simulink model "Ld_Lq_realised_inverter"  (R2021b)
settings: Solver=ode23tb  StartTime=0.0  StopTime=0.05  MaxStep=1e-6  RelTol=1e-3  EnableMultiTasking=on
libraries: spsMosfetLib x6, spsCurrentMeasurementLib x5, spsRMSLib x5, spsVoltageMeasurementLib x4, spsSeriesRLCBranchLib x2, spsMeanLib x2, spsDCVoltageSourceLib x1, spsThreePhaseSeriesRLCBranchLib x1, simulink x1, spspowerguiLib x1
settings Model: SimulationMode=accelerator  Creator=Алексей  LastModifiedBy=Len_comp
settings SolverCC: ZeroCrossControl=DisableAll  ZeroCrossAlgorithm=Adaptive  AlgebraicLoopSolver=TrustRegion
settings DataIOCC: SaveFormat=Array  SaveOutput=off  SignalLogging=off  DSMLogging=off  SaveTime=off  ReturnWorkspaceOutputs=off
settings OptimizationCC: LifeSpan=inf
settings DebuggingCC: UnderspecifiedInitializationDetection=Classic  MergeDetectMultiDrivingBlocksExec=none  SolverPrmCheckMsg=warning  AllowSymbolicDim=off  SFUnexpectedBacktrackingDiag=warning  SFNoUnconditionalDefaultTransitionDiag=warning  SFExecutionAtInitializationDiag=none  SFMachineParentedDataDiag=warning  ArithmeticOperatorsInVariantConditions=warning
settings HardwareCC: ProdBitPerPointer=32  ProdBitPerSizeT=32  ProdBitPerPtrDiffT=32  ProdLargestAtomicFloat=None  ProdIntDivRoundTo=Undefined  ProdEndianess=Unspecified  ProdWordSize=32  ProdHWDeviceType=32-bit Generic
settings ModelReferenceCC: PropagateSignalLabelsOutOfModel=off
settings SFSimCC: SimUseLocalCustomCode=off  CustomCodeUndefinedFunction=UseInterfaceOnly
settings RTWCC: RTWUseLocalCustomCode=off
settings CodeAppCC: StateflowObjectComments=on
settings GRTTargetCC: TargetLangStandard=C89/C90 (ANSI)  RTWCAPISignals=on  RTWCAPIParams=on
settings ConfigComp: CovMetricSettings=dw  CovSaveCumulativeToWorkspaceVar=on  CovSaveSingleToWorkspaceVar=on  CovExternalEMLEnable=off  CovSFcnEnable=off
settings SimscapeCC: SimscapeNormalizeSystem=off

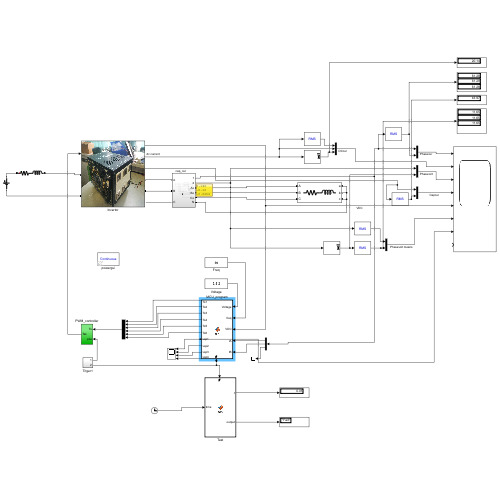
[thumbnail: Simulink's stored preview of the top-level diagram]
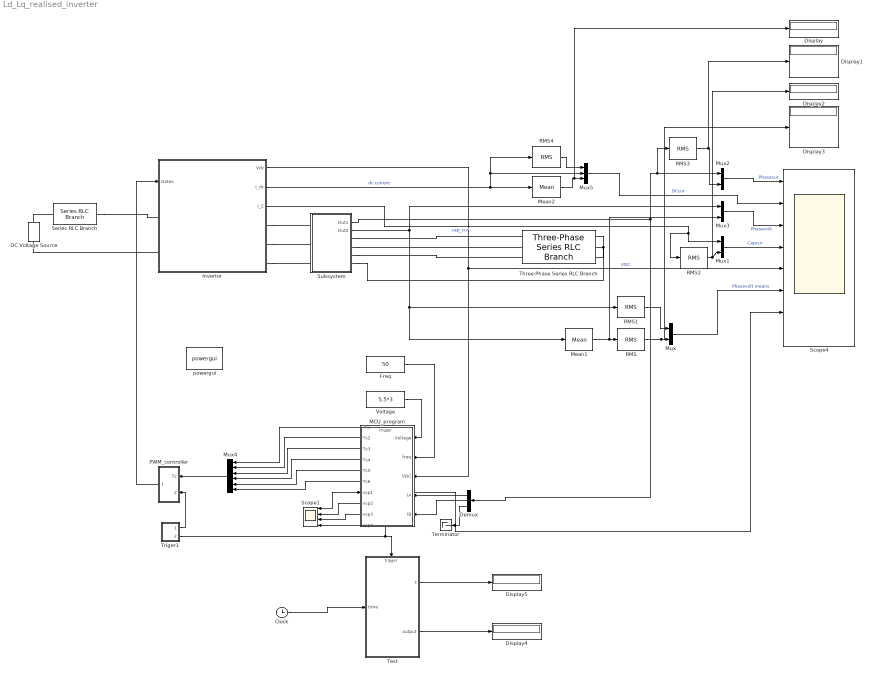
== system Ld_Lq_realised_inverter ==
  Clock : Clock
  DC Voltage Source : spsDCVoltageSourceLib/DC Voltage Source  Amplitude=100  Measurements=None
  Demux : Demux  Outputs=3
  Display{,1..5} (6 alike) : Display
      Display settings: Decimation=3
  Freq : Constant  Value=50
  Invertor : Subsystem
      mask Display: image('$imagefile'); % Use "Edit Image" on toolstrip to change.
  MCU_program : MATLAB Function  TreatAsAtomicUnit=on
  Mean1 : spsMeanLib/Mean  Freq=10000  Vinit=0  Ts=0
  Mean2 : spsMeanLib/Mean  Freq=1000  Vinit=0  Ts=0
  Mux{,1..3} (4 alike) : Mux  Inputs=2
  Mux4 : Mux  Inputs=6
  Mux5 : Mux  Inputs=3
  PWM_controller : Subsystem
  RMS{,1..4} (5 alike) : spsRMSLib/RMS  TrueRMS=on  Freq=50  RMSInit=0  Ts=0
  Scope1 : Scope  NumInputPorts=4
  Scope4 : Scope  NumInputPorts=8
  Series RLC Branch : spsSeriesRLCBranchLib/Series RLC Branch  LConnTagsString=__new0  RConnTagsString=__new0  BranchType=RL  Resistance=1e-3  Inductance=1e-6  SetiL0=off  InitialCurrent=0  Capacitance=1e-6  Setx0=off  InitialVoltage=0  Measurements=None
  Subsystem : Subsystem
  Terminator : Terminator
  Test : MATLAB Function  TreatAsAtomicUnit=on
  Three-Phase Series RLC Branch : spsThreePhaseSeriesRLCBranchLib/Three-Phase Series RLC Branch  LConnTagsString=A|B|C  RConnTagsString=A|B|C  BranchType=RL  Resistance=0.06*3  Inductance=(60e-6)*3  Capacitance=1e-6  Measurements=None
  Triger1 : Subsystem
  Voltage : Constant  Value=5.5*3
  powergui : spspowerguiLib/powergui  Priority=1  SimulationMode=Continuous  SampleTime=50e-6  frequency=60  Iterations=50  frequencyindice=0  Pbase=100e6  ErrMax=1e-4  UnitsV=kV  UnitsW=MW  buscounter=0  FunctionMessages=off  echomessages=off  EnableUseOfTLC=off  CurrentSourceSwitches=on  DisableSnubberDevices=off  DisableRonSwitches=off  DisableVfSwitches=off  DisplayEquations=off  AutomaticDiscreteSolvers=off  SolverType=Tustin  Interpol=off  ExternalGateDelay=off  methode=off  Ts=0  x0status=blocks  SPID=off  SwTol=0  HookPort=off  NonlinearTolerance=1e-4  nMaxIteration=100  ContinueOnMaxIteration=off  RestoreLinks=warning  ResistiveCurrentMeasurement=off  Frange=[0:2:500]  Ylog=off  Xlog=on  ShowGrid=off  save=off  variable=ZData  structure=SD2  ZoomFFT=on  StartTime=0.7  cycles=10  DisplayStyle=4  fundamental=382  FreqAxis=off  MaxFrequency=50000  frequencyindicesteady=1  RmsSteady=1  display=off
  wires:
  MCU_program/8(vsp2) -> Scope1/2
  MCU_program/9(vsp3) -> Scope1/3
  MCU_program/7(vsp1) -> Scope1/1, Scope4/7
  MCU_program/10(vsp4) -> Scope1/4
  Voltage/1 -> MCU_program/1(Voltage)
  MCU_program/6(Ts6) -> Mux4/6
  MCU_program/5(Ts5) -> Mux4/5
  MCU_program/4(Ts4) -> Mux4/4
  MCU_program/3(Ts3) -> Mux4/3
  Triger1/1(1) -> PWM_controller/2(pila)
  PWM_controller/1(Tss) -> Invertor/1(Gates)
  MCU_program/1(Ts1) -> Mux4/1
  Mux4/1 -> PWM_controller/1(Ts)
  Triger1/2(2) -> Test/Trigger, MCU_program/Trigger
  MCU_program/2(Ts2) -> Mux4/2
  Invertor/1(Vdc) -> MCU_program/3(VDC), Scope4/5  "VDC"
  Invertor/2(I_dc) -> Mux5/2, RMS4/1, Mean2/1  "dc current"
  Subsystem/1(Out1) -> RMS3/1, Mux2/1, Demux/1
  Subsystem/2(Out2) -> Mux3/1, Mean1/1, RMS1/1
  Freq/1 -> MCU_program/2(freq)
  Invertor/3(I_C) -> RMS2/1, Mux1/1  "cap_cur"
  Demux/3 -> Terminator/1
  Demux/1 -> MCU_program/4(IA)
  Demux/2 -> MCU_program/5(IB)
  RMS1/1 -> Mux/1
  Mean1/1 -> Mux3/2, RMS/1
  Mux/1 -> Scope4/6  "Phasevolt means"
  RMS/1 -> Display3/1, Mux/2
  RMS2/1 -> Display2/1, Mux1/2
  Mux1/1 -> Scope4/4  "Capcur"
  Mux2/1 -> Scope4/1  "Phasecur"
  RMS3/1 -> Display1/1, Mux2/2
  Mux3/1 -> Scope4/3  "Phasevolt"
  Mean2/1 -> Display/1, Mux5/3
  RMS4/1 -> Mux5/1
  Mux5/1 -> Scope4/2  "DCcur"
  Test/2(output) -> Display4/1
  Clock/1 -> Test/1(time)
  Test/1(t) -> Display5/1
  connections:
  Three-Phase Series RLC Branch/RConn1 -- Subsystem/RConn4 -- Three-Phase Series RLC Branch/RConn3 -- Three-Phase Series RLC Branch/RConn2
  Invertor/RConn1 -- Subsystem/LConn1
  Subsystem/RConn1 -- Three-Phase Series RLC Branch/LConn1
  Invertor/RConn2 -- Subsystem/LConn2
  Subsystem/RConn2 -- Three-Phase Series RLC Branch/LConn2
  Invertor/RConn3 -- Subsystem/LConn3
  Subsystem/RConn3 -- Three-Phase Series RLC Branch/LConn3
  DC Voltage Source/RConn1 -- Series RLC Branch/LConn1
  Series RLC Branch/RConn1 -- Invertor/LConn1
  DC Voltage Source/LConn1 -- Invertor/LConn2

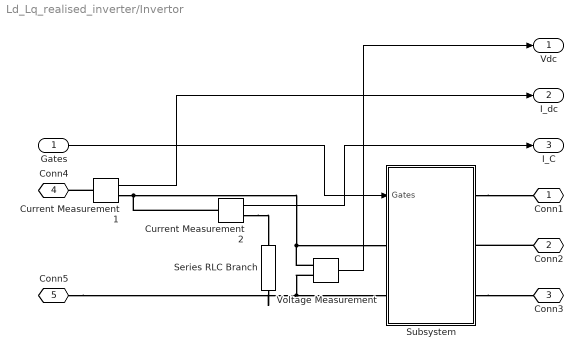
== system Ld_Lq_realised_inverter/Invertor ==
  Gates : Inport
  Current Measurement1 : spsCurrentMeasurementLib/Current Measurement  PhasorSimulation=off  OutputType=Complex  PSBequivalent=0
  Current Measurement2 : spsCurrentMeasurementLib/Current Measurement  PhasorSimulation=off  OutputType=Complex  PSBequivalent=0
  Series RLC Branch : spsSeriesRLCBranchLib/Series RLC Branch  LConnTagsString=__new0  RConnTagsString=__new0  BranchType=C  Resistance=1  Inductance=1e-3  SetiL0=off  InitialCurrent=0  Capacitance=1000e-6  Setx0=on  InitialVoltage=100  Measurements=None
  Subsystem : Subsystem
  Voltage Measurement : spsVoltageMeasurementLib/Voltage Measurement  PhasorSimulation=off  OutputType=Complex  PSBequivalent=0
  Conn1 : PMIOPort  Side=Right
  Conn2 : PMIOPort  Port=2  Side=Right
  Conn3 : PMIOPort  Port=3  Side=Right
  Conn4 : PMIOPort  Port=4  Side=Left
  Conn5 : PMIOPort  Port=5  Side=Left
  Vdc : Outport  VectorParamsAs1DForOutWhenUnconnected=off
  I_dc : Outport  Port=2  VectorParamsAs1DForOutWhenUnconnected=off
  I_C : Outport  Port=3  VectorParamsAs1DForOutWhenUnconnected=off
  wires:
  Voltage Measurement/1 -> Vdc/1
  Gates/1 -> Subsystem/1(Gates)
  Current Measurement1/1 -> I_dc/1
  Current Measurement2/1 -> I_C/1
  connections:
  Current Measurement1/LConn1 -- Conn4/RConn1
  Voltage Measurement/LConn2 -- Conn5/RConn1 -- Series RLC Branch/RConn1 -- Subsystem/LConn2
  Subsystem/RConn1 -- Conn1/RConn1
  Conn2/RConn1 -- Subsystem/RConn2
  Subsystem/RConn3 -- Conn3/RConn1
  Current Measurement1/RConn1 -- Current Measurement2/LConn1 -- Voltage Measurement/LConn1 -- Subsystem/LConn1
  Current Measurement2/RConn1 -- Series RLC Branch/LConn1

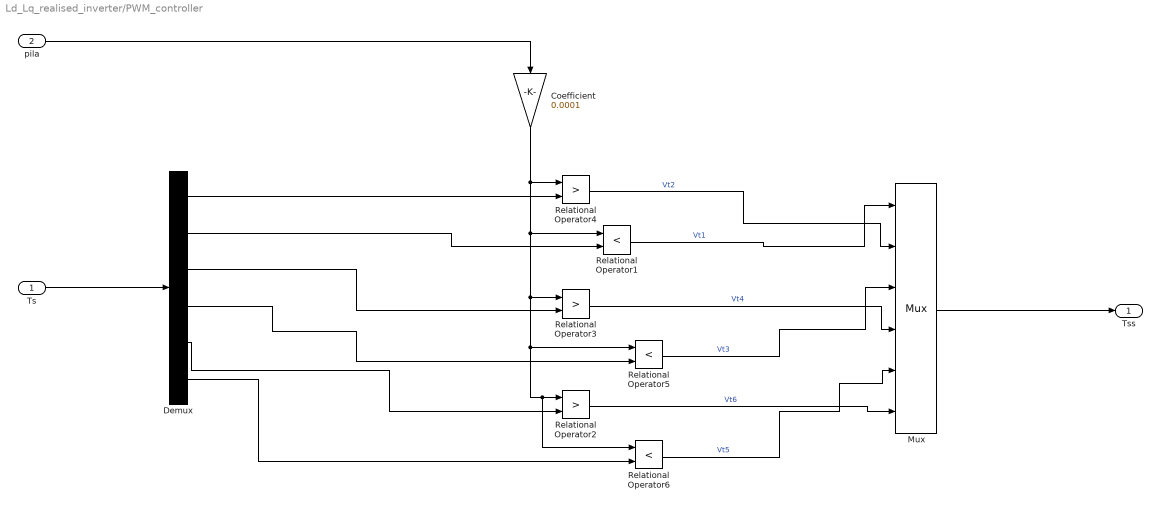
== system Ld_Lq_realised_inverter/PWM_controller ==
  Ts : Inport
  pila : Inport  Port=2
  Coefficient : Gain  Gain=0.0001
  Demux : Demux  Outputs=6
  Mux : Mux  Inputs=6
  Relational Operator1 : RelationalOperator  Operator=<  OutDataTypeStr=boolean  RndMeth=Nearest
  Relational Operator2 : RelationalOperator  Operator=>  OutDataTypeStr=boolean  RndMeth=Nearest
  Relational Operator3 : RelationalOperator  Operator=>  OutDataTypeStr=boolean  RndMeth=Nearest
  Relational Operator4 : RelationalOperator  Operator=>  OutDataTypeStr=boolean  RndMeth=Nearest
  Relational Operator5 : RelationalOperator  Operator=<  OutDataTypeStr=boolean  RndMeth=Nearest
  Relational Operator6 : RelationalOperator  Operator=<  OutDataTypeStr=boolean  RndMeth=Nearest
  Tss : Outport  VectorParamsAs1DForOutWhenUnconnected=off
  wires:
  Relational Operator4/1 -> Mux/2  "Vt2"
  Demux/3 -> Relational Operator3/2
  Demux/5 -> Relational Operator2/2
  Relational Operator3/1 -> Mux/4  "Vt4"
  Relational Operator2/1 -> Mux/6  "Vt6"
  Ts/1 -> Demux/1
  Coefficient/1 -> Relational Operator1/1, Relational Operator3/1, Relational Operator5/1, Relational Operator6/1, Relational Operator2/1, Relational Operator4/1
  Relational Operator1/1 -> Mux/1  "Vt1"
  Relational Operator5/1 -> Mux/3  "Vt3"
  Relational Operator6/1 -> Mux/5  "Vt5"
  Demux/2 -> Relational Operator1/2
  Demux/4 -> Relational Operator5/2
  Demux/6 -> Relational Operator6/2
  Demux/1 -> Relational Operator4/2
  pila/1 -> Coefficient/1
  Mux/1 -> Tss/1

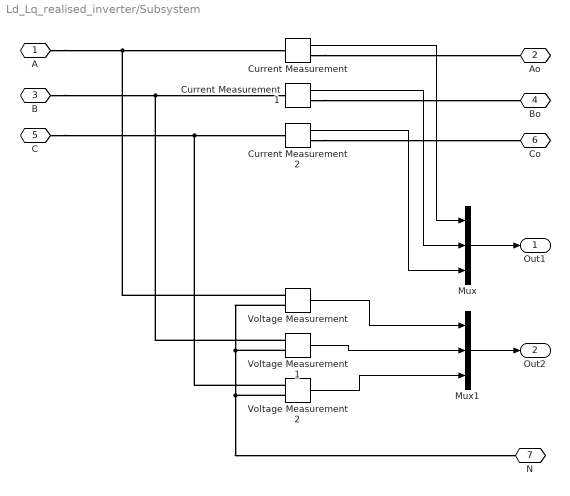
== system Ld_Lq_realised_inverter/Subsystem ==
  Current Measurement : spsCurrentMeasurementLib/Current Measurement  PhasorSimulation=off  OutputType=Complex  PSBequivalent=0
  Current Measurement1 : spsCurrentMeasurementLib/Current Measurement  PhasorSimulation=off  OutputType=Complex  PSBequivalent=0
  Current Measurement2 : spsCurrentMeasurementLib/Current Measurement  PhasorSimulation=off  OutputType=Complex  PSBequivalent=0
  Mux : Mux  Inputs=3
  Mux1 : Mux  Inputs=3
  Voltage Measurement : spsVoltageMeasurementLib/Voltage Measurement  PhasorSimulation=off  OutputType=Complex  PSBequivalent=0
  Voltage Measurement1 : spsVoltageMeasurementLib/Voltage Measurement  PhasorSimulation=off  OutputType=Complex  PSBequivalent=0
  Voltage Measurement2 : spsVoltageMeasurementLib/Voltage Measurement  PhasorSimulation=off  OutputType=Complex  PSBequivalent=0
  A : PMIOPort  Side=Left
  Ao : PMIOPort  Port=2  Side=Right
  B : PMIOPort  Port=3  Side=Left
  Bo : PMIOPort  Port=4  Side=Right
  C : PMIOPort  Port=5  Side=Left
  Co : PMIOPort  Port=6  Side=Right
  N : PMIOPort  Port=7  Side=Right
  Out1 : Outport
  Out2 : Outport  Port=2
  wires:
  Mux1/1 -> Out2/1
  Current Measurement1/1 -> Mux/2
  Current Measurement2/1 -> Mux/3
  Voltage Measurement2/1 -> Mux1/3
  Voltage Measurement1/1 -> Mux1/2
  Voltage Measurement/1 -> Mux1/1
  Current Measurement/1 -> Mux/1
  Mux/1 -> Out1/1
  connections:
  Voltage Measurement2/LConn1 -- Current Measurement2/LConn1 -- C/RConn1
  Voltage Measurement1/LConn2 -- Voltage Measurement/LConn2 -- N/RConn1 -- Voltage Measurement2/LConn2
  Voltage Measurement1/LConn1 -- Current Measurement1/LConn1 -- B/RConn1
  Voltage Measurement/LConn1 -- Current Measurement/LConn1 -- A/RConn1
  Current Measurement2/RConn1 -- Co/RConn1
  Current Measurement/RConn1 -- Ao/RConn1
  Current Measurement1/RConn1 -- Bo/RConn1

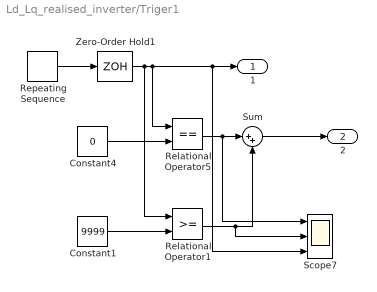
== system Ld_Lq_realised_inverter/Triger1 ==
  Constant1 : Constant  Value=9999
  Constant4 : Constant  Value=0
  Relational Operator1 : RelationalOperator  OutDataTypeStr=boolean  RndMeth=Nearest
  Relational Operator5 : RelationalOperator  Operator===  OutDataTypeStr=boolean  RndMeth=Nearest
  Repeating Sequence : simulink/Sources/Repeating Sequence  rep_seq_t=[0 10e-5 20e-5]  rep_seq_y=[0 10000 0]
  Scope7 : Scope  NumInputPorts=3
  Sum : Sum  Inputs=|++
  Zero-Order Hold1 : ZeroOrderHold  SampleTime=2.5e-8
  1 : Outport  VectorParamsAs1DForOutWhenUnconnected=off
  2 : Outport  Port=2  VectorParamsAs1DForOutWhenUnconnected=off
  wires:
  Zero-Order Hold1/1 -> Relational Operator1/1, Relational Operator5/1, Scope7/3, 1/1
  Repeating Sequence/1 -> Zero-Order Hold1/1
  Constant4/1 -> Relational Operator5/2
  Sum/1 -> 2/1
  Constant1/1 -> Relational Operator1/2
  Relational Operator5/1 -> Scope7/1, Sum/1
  Relational Operator1/1 -> Scope7/2, Sum/2

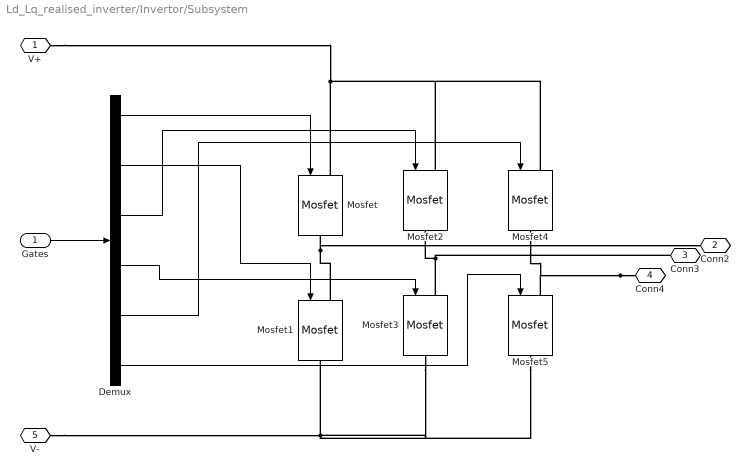
== system Ld_Lq_realised_inverter/Invertor/Subsystem ==
  Gates : Inport
  Demux : Demux  Outputs=6
  Mosfet{,1..5} (6 alike) : spsMosfetLib/Mosfet  Ron=2e-3  Lon=0  Rd=0.01  Vfd=0  IC=0  Rs=1e5  Cs=inf  Measurements=off
  V+ : PMIOPort  Side=Left
  Conn2 : PMIOPort  Port=2  Side=Right
  Conn3 : PMIOPort  Port=3  Side=Right
  Conn4 : PMIOPort  Port=4  Side=Right
  V- : PMIOPort  Port=5  Side=Left
  wires:
  Demux/4 -> Mosfet3/1
  Demux/2 -> Mosfet1/1
  Demux/5 -> Mosfet4/1
  Demux/3 -> Mosfet2/1
  Demux/6 -> Mosfet5/1
  Demux/1 -> Mosfet/1
  Gates/1 -> Demux/1
  connections:
  Conn4/RConn1 -- Mosfet5/LConn1 -- Mosfet4/RConn1
  V-/RConn1 -- Mosfet1/RConn1 -- Mosfet5/RConn1 -- Mosfet3/RConn1
  Conn3/RConn1 -- Mosfet2/RConn1 -- Mosfet3/LConn1
  V+/RConn1 -- Mosfet/LConn1 -- Mosfet4/LConn1 -- Mosfet2/LConn1
  Mosfet1/LConn1 -- Conn2/RConn1 -- Mosfet/RConn1

== matlab function Ld_Lq_realised_inverter/Test ==
  data: t output; time input; output output
  events: trigger input RISING_EDGE_EVENT
function [t, output]  = fcn(time)
persistent cnt 
if isempty(cnt)
    cnt = 0;
end
t = time;

output = "Fail!";

cnt = cnt + 1;
return;

== matlab function Ld_Lq_realised_inverter/MCU_program ==
  data: Voltage input; freq input; Ts1 output; Ts2 output; Ts3 output; Ts4 output; Ts5 output; Ts6 output; vsp1 output; vsp2 output; vsp3 output; vsp4 output; VDC input; IA input; IB input
  events: trigger input RISING_EDGE_EVENT
function [Ts1,Ts2,Ts3,Ts4,Ts5,Ts6,vsp1,vsp2,vsp3,vsp4] = fcn(Voltage, freq,VDC,IA,IB)
%время 1/2 ШИМ периода
dt=100e-6;

dead_time=0;

persistent teta
if(isempty(teta))
    teta = 0;
end

teta = teta + 2 * pi * freq * dt;
teta = mod(teta,2*pi);
Ua0=Voltage*cos(teta);
Ub0=Voltage*sin(teta);

vrefa=sqrt(Ua0^2+Ub0^2);

vphase=acos(Ua0/vrefa)*sign(Ub0)+(sign(Ub0)-1)*(-pi);

if(vrefa>(2/3)*VDC)
vrefa = 2/3*VDC;
end

vsp1=teta;
vsp2=sin(pi);
vsp3=sin(90);%wzad-omeg;
vsp4=0;


%алгоритм формирования векторной ШИМ  мертвым веменем dead [мкс]

dead_time=dead_time/(dt*1e6);
a=vphase;
v2=vrefa*1.5;
if a>=0 && a<pi/3 
    n=1;
elseif  a>=pi/3 && a<2*pi/3 
    n=2;
elseif  a>=2*pi/3 && a<pi 
    n=3;
elseif  a>=pi && a<4*pi/3 
    n=4;
elseif  a>=4*pi/3 && a<5*pi/3 
    n=5;
else n=6;

end

a_cor=a-(n-1)*pi/3;

T1 = (v2/VDC)*sin(pi/3-a_cor)/sin(pi/3);
T2 = (v2/VDC)*sin(a_cor)/sin(pi/3);
T0=1-T1-T2;
Ta1=0; Ta3=0; Ta5=0; 
switch n
    case 1
        
        Ta1=T1+T2+T0/2;
        
        Ta3=T2+T0/2;
       
        Ta5=T0/2;
       
    case 2
        
        Ta1=T1+T0/2;
        
        Ta3=T1+T2+T0/2;
    
        Ta5=T0/2;       
        
    case 3
        
        Ta1=T0/2;
       
        Ta3=T1+T2+T0/2;
       
        Ta5=T2+T0/2;    
        
    case 4
        
        Ta1=T0/2;
       
        Ta3=T1+T0/2;
       
        Ta5=T1+T2+T0/2;   
       
    case 5
        
        Ta1=T2+T0/2;
        
        Ta3=T0/2;
        
        Ta5=T1+T2+T0/2;     
        
    case 6
        
        Ta1=T1+T2+T0/2;
        
        Ta3=T0/2;
     
        Ta5=T1+T0/2;    
        
end;


Ts1=(Ta1)+dead_time/2; 
Ts3=(Ta3)+dead_time/2; 
Ts5=(Ta5)+dead_time/2;
Ts2=(Ta1)-dead_time/2; 
Ts4=(Ta3)-dead_time/2; 
Ts6=(Ta5)-dead_time/2;


if (IA>0) 
    Ts1=Ts1+dead_time/2;
    Ts2=Ts2+dead_time/2;
else
    Ts1=Ts1-dead_time/2;
    Ts2=Ts2-dead_time/2;           
end;
if (IB>0) 
    Ts3=Ts3+dead_time/2;
    Ts4=Ts4+dead_time/2;
else
    Ts3=Ts3-dead_time/2;
    Ts4=Ts4-dead_time/2; 
end;  
if ((-IA-IB)>0) 
    Ts5=Ts5+dead_time/2;
    Ts6=Ts6+dead_time/2;
else
    Ts5=Ts5-dead_time/2;
    Ts6=Ts6-dead_time/2;           
end;


return;



return;
